simulink model "AD_AlfBet"  (Simulink 5.0)
settings: Solver=ode45  StartTime=0.0  StopTime=0.4  RelTol=1e-3
settings Model: LastModifiedBy=papa

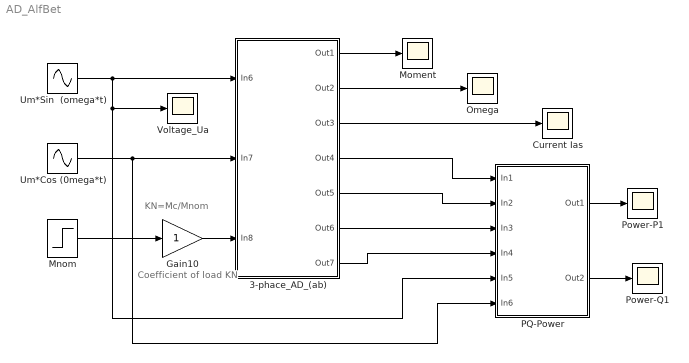
== system AD_AlfBet ==
  note: Coefficient of load
      | KN
  note: KN=Mc/Mnom
  " 3-phace_AD_(ab)" : Subsystem
  Current Ias : Scope
      settings: TickLabels=on  TimeRange=0.5  YMin=-15  YMax=15  SaveName=ScopeData2  DataFormat=Array
  Gain10 : Gain  SaturateOnIntegerOverflow=on
  Mnom : Step  Time=0.06  Before=0.0  After=17  SampleTime=0
  Moment : Scope
      settings: TickLabels=on  TimeRange=80  YMin=-1  YMax=2  DataFormat=Array
  Omega : Scope
      settings: TickLabels=on  TimeRange=0.5  YMin=0  YMax=200  DataFormat=Array
  PQ-Power : Subsystem
  Power-P1 : Scope
      settings: TickLabels=on  TimeRange=0.5  YMin=-15  YMax=15  SaveName=ScopeData4  DataFormat=Array
  Power-Q1 : Scope
      settings: TickLabels=on  TimeRange=0.5  YMin=-15  YMax=15  SaveName=ScopeData5  DataFormat=Array
  Um*Cos (0mega*t) : Sin  Amplitude=311  Frequency=314  Phase=-pi/2  SampleTime=0
  Um*Sin  (omega*t) : Sin  Amplitude=311  Frequency=314  SampleTime=0
  Voltage_Ua : Scope
      settings: TickLabels=on  TimeRange=0.5  YMin=-15  YMax=15  SaveName=ScopeData3  DataFormat=Array
  wires:
  " 3-phace_AD_(ab)"/1(Out1) -> Moment/1
  " 3-phace_AD_(ab)"/2(Out2) -> Omega/1
  " 3-phace_AD_(ab)"/3(Out3) -> Current Ias/1
  Um*Cos (0mega*t)/1 -> PQ-Power/6(In6), " 3-phace_AD_(ab)"/2(In7)
  " 3-phace_AD_(ab)"/4(Out4) -> PQ-Power/1(In1)
  " 3-phace_AD_(ab)"/5(Out5) -> PQ-Power/2(In2)
  " 3-phace_AD_(ab)"/6(Out6) -> PQ-Power/3(In3)
  Um*Sin  (omega*t)/1 -> " 3-phace_AD_(ab)"/1(In6), Voltage_Ua/1, PQ-Power/5(In5)
  PQ-Power/1(Out1) -> Power-P1/1
  PQ-Power/2(Out2) -> Power-Q1/1
  " 3-phace_AD_(ab)"/7(Out7) -> PQ-Power/4(In4)
  Mnom/1 -> Gain10/1
  Gain10/1 -> " 3-phace_AD_(ab)"/3(In8)

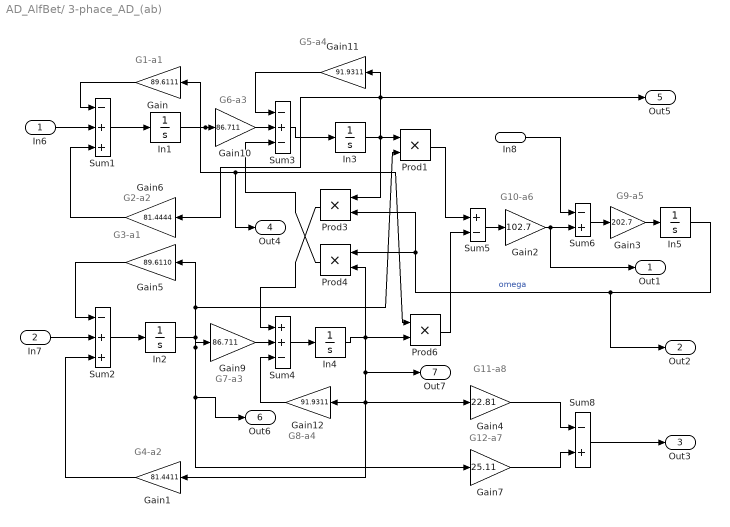
== system AD_AlfBet/ 3-phace_AD_(ab) ==
  note: G1-a1
  note: G2-a2
  note: G3-a1
  note: G4-a2
  note: G10-a6
  note: G9-a5
  note: G6-a3
  note: G7-a3
  note: G8-a4
  note: G5-a4
  note: G11-a8
  note: G12-a7
  In6 : Inport
  In7 : Inport  Port=2
  In8 : Inport  Port=3
  "  Prod1" : Product  SaturateOnIntegerOverflow=on  InputSameDT=on
  Gain : Gain  Orientation=left  Gain=89.6111  SaturateOnIntegerOverflow=on
  Gain1 : Gain  Orientation=left  Gain=81.4411  SaturateOnIntegerOverflow=on
  Gain10 : Gain  Gain=86.711  SaturateOnIntegerOverflow=on
  Gain11 : Gain  Orientation=left  Gain=91.9311  SaturateOnIntegerOverflow=on
  Gain12 : Gain  Orientation=left  Gain=91.9311  SaturateOnIntegerOverflow=on
  Gain2 : Gain  Gain=102.7  SaturateOnIntegerOverflow=on
  Gain3 : Gain  Gain=202.7  SaturateOnIntegerOverflow=on
  Gain4 : Gain  Gain=22.81  SaturateOnIntegerOverflow=on
  Gain5 : Gain  Orientation=left  Gain=89.6110  SaturateOnIntegerOverflow=on
  Gain6 : Gain  Orientation=left  Gain=81.4444  SaturateOnIntegerOverflow=on
  Gain7 : Gain  Gain=25.11  SaturateOnIntegerOverflow=on
  Gain9 : Gain  Gain=86.711  SaturateOnIntegerOverflow=on
  In{1..5} (5 alike) : Integrator
  Prod3 : Product  Orientation=left  SaturateOnIntegerOverflow=on  InputSameDT=on
  Prod4 : Product  Orientation=left  SaturateOnIntegerOverflow=on  InputSameDT=on
  Prod6 : Product  SaturateOnIntegerOverflow=on  InputSameDT=on
  Sum1 : Sum  Inputs=-++  SaturateOnIntegerOverflow=on  InputSameDT=on
  Sum2 : Sum  Inputs=-++  SaturateOnIntegerOverflow=on  InputSameDT=on
  Sum3 : Sum  Inputs=-+-  SaturateOnIntegerOverflow=on  InputSameDT=on
  Sum4 : Sum  Inputs=++-  SaturateOnIntegerOverflow=on  InputSameDT=on
  Sum5 : Sum  Inputs=+-  SaturateOnIntegerOverflow=on  InputSameDT=on
  Sum6 : Sum  Inputs=-+  SaturateOnIntegerOverflow=on  InputSameDT=on
  Sum8 : Sum  Inputs=-+  SaturateOnIntegerOverflow=on  InputSameDT=on
  Out1 : Outport
  Out2 : Outport  Port=2
  Out3 : Outport  Port=3
  Out4 : Outport  Port=4
  Out5 : Outport  Port=5
  Out6 : Outport  Port=6
  Out7 : Outport  Port=7
  wires:
  Gain/1 -> Sum1/1
  Sum2/1 -> In2/1
  In4/1 -> Prod4/2, Prod6/2, Gain1/1, Gain12/1, Gain4/1, Out7/1
  In3/1 -> Prod3/1, "  Prod1"/1, Gain6/1, Gain11/1, Out5/1
  Prod6/1 -> Sum5/2
  Gain3/1 -> In5/1
  In8/1 -> Sum6/1
  "  Prod1"/1 -> Sum5/1
  Sum3/1 -> In3/1
  Sum5/1 -> Gain2/1
  Sum1/1 -> In1/1
  In2/1 -> "  Prod1"/2, Gain5/1, Gain9/1, Gain7/1, Out6/1
  In1/1 -> Gain10/1, Gain/1, Prod6/1, Out4/1
  Gain10/1 -> Sum3/2
  Gain9/1 -> Sum4/2
  Gain5/1 -> Sum2/1
  Prod4/1 -> Sum3/3
  Prod3/1 -> Sum4/1
  Gain2/1 -> Sum6/2, Out1/1
  Gain11/1 -> Sum3/1
  Gain12/1 -> Sum4/3
  In5/1 -> Prod3/2, Prod4/1, Out2/1  "omega"
  Sum4/1 -> In4/1
  Gain7/1 -> Sum8/2
  Gain4/1 -> Sum8/1
  Gain6/1 -> Sum1/3
  Gain1/1 -> Sum2/3
  In7/1 -> Sum2/2
  In6/1 -> Sum1/2
  Sum8/1 -> Out3/1
  Sum6/1 -> Gain3/1

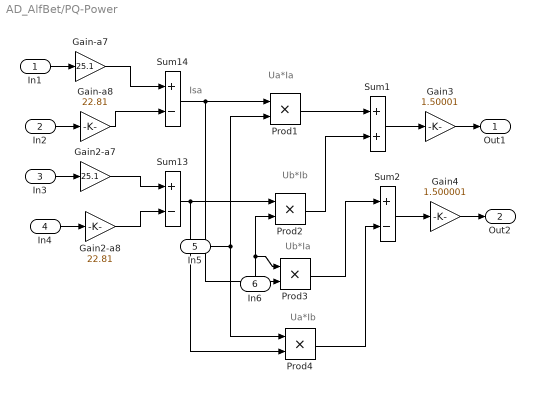
== system AD_AlfBet/PQ-Power ==
  note: Isa
  note: Ua*Ia
  note: Ub*Ib
  note: Ub*Ia
  note: Ua*Ib
  In1 : Inport
  In2 : Inport  Port=2
  In3 : Inport  Port=3
  In4 : Inport  Port=4
  In5 : Inport  Port=5
  In6 : Inport  Orientation=up  Port=6
    Prod{1..4} (4 alike) : Product  SaturateOnIntegerOverflow=on  InputSameDT=on
  Gain-a7 : Gain  Gain=25.1  SaturateOnIntegerOverflow=on
  Gain-a8 : Gain  Gain=22.81  SaturateOnIntegerOverflow=on
  Gain2-a7 : Gain  Gain=25.1  SaturateOnIntegerOverflow=on
  Gain2-a8 : Gain  Gain=22.81  SaturateOnIntegerOverflow=on
  Gain3 : Gain  Gain=1.50001  SaturateOnIntegerOverflow=on
  Gain4 : Gain  Gain=1.500001  SaturateOnIntegerOverflow=on
  Sum1 : Sum  SaturateOnIntegerOverflow=on  InputSameDT=on
  Sum13 : Sum  Inputs=+-  SaturateOnIntegerOverflow=on  InputSameDT=on
  Sum14 : Sum  Inputs=+-  SaturateOnIntegerOverflow=on  InputSameDT=on
  Sum2 : Sum  Inputs=+-  SaturateOnIntegerOverflow=on  InputSameDT=on
  Out1 : Outport
  Out2 : Outport  Port=2
  wires:
  Gain-a7/1 -> Sum14/1
  Gain-a8/1 -> Sum14/2
  Gain2-a7/1 -> Sum13/1
  Gain2-a8/1 -> Sum13/2
  Sum14/1 -> "  Prod1"/1, "  Prod3"/2
  Sum13/1 -> "  Prod2"/1, "  Prod4"/2
  "  Prod1"/1 -> Sum1/1
  "  Prod2"/1 -> Sum1/2
  Sum1/1 -> Gain3/1
  "  Prod3"/1 -> Sum2/1
  "  Prod4"/1 -> Sum2/2
  Sum2/1 -> Gain4/1
  In5/1 -> "  Prod1"/2, "  Prod4"/1
  In6/1 -> "  Prod2"/2, "  Prod3"/1
  In1/1 -> Gain-a7/1
  In2/1 -> Gain-a8/1
  Gain3/1 -> Out1/1
  In3/1 -> Gain2-a7/1
  Gain4/1 -> Out2/1
  In4/1 -> Gain2-a8/1
